simulink model "ss2tf_model"  (R2018b)
settings: Solver=VariableStepAuto  StartTime=0.0  StopTime=600  RelTol=1e-3
undefined symbols (not defined in the file or in its folder): filteredInvTF, heave, seaWave, SS_full, surge
settings Model: Creator=user  LastModifiedBy=user

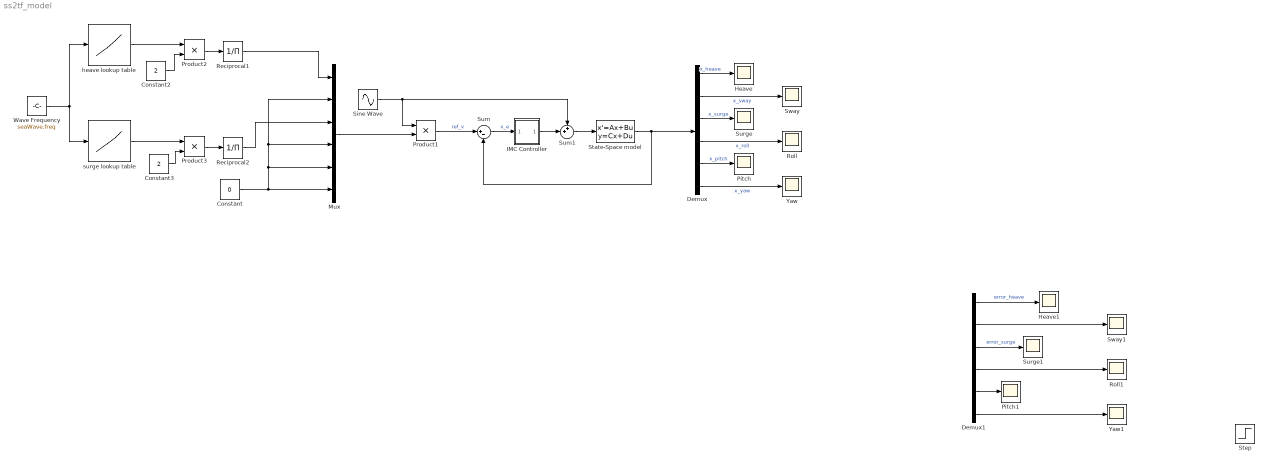
== system ss2tf_model ==
  Constant : Constant  Value=0
  Constant2 : Constant  Value=2
  Constant3 : Constant  Value=2
  Demux : Demux  Outputs=6
  Demux1 : Demux  Outputs=6
  Heave : Scope
  Heave1 : Scope
  IMC Controller : Subsystem
      mask Display: fprintf("K")
  Mux : Mux  Inputs=6
  Pitch : Scope
  Pitch1 : Scope
  Product1 : Product
  Product2 : Product
  Product3 : Product
  Reciprocal1 : Product  Inputs=/
  Reciprocal2 : Product  Inputs=/
  Roll : Scope
  Roll1 : Scope
  Sine Wave : Sin  Amplitude=seaWave.amp  Frequency=seaWave.freq  SampleTime=0
  State-Space model : StateSpace  A=SS_full.A  B=SS_full.B  C=SS_full.C  D=SS_full.D  InitialCondition=0
  Step : Step  Time=20  SampleTime=0
  Sum : Sum  Inputs=|+-
  Sum1 : Sum  Inputs=++|
  Surge : Scope
  Surge1 : Scope
  Sway : Scope
  Sway1 : Scope
  Wave Frequency : Constant  Value=seaWave.freq
  Yaw : Scope
  Yaw1 : Scope
  heave lookup table : Lookup_n-D  NumberOfTableDimensions=1  BreakpointsForDimension1=heave.freq  Table=heave.amp  InternalRulePriority=Speed  RndMeth=Simplest  InputSameDT=on
  surge lookup table : Lookup_n-D  NumberOfTableDimensions=1  BreakpointsForDimension1=surge.freq  Table=surge.amp  InternalRulePriority=Speed  RndMeth=Simplest  InputSameDT=on
  wires:
  Wave Frequency/1 -> heave lookup table/1, surge lookup table/1
  Constant/1 -> Mux/2, Mux/4, Mux/5, Mux/6
  Mux/1 -> Product1/2
  Product1/1 -> Sum/1  "ref_v"
  Sine Wave/1 -> Sum1/1, Product1/1
  Demux/1 -> Heave/1  "x_heave"
  Demux/3 -> Surge/1  "x_surge"
  Demux/5 -> Pitch/1  "x_pitch"
  Sum1/1 -> State-Space model/1
  Sum/1 -> IMC Controller/1(x_e)  "x_e"
  IMC Controller/1(control signal) -> Sum1/2
  Demux/2 -> Sway/1  "x_sway"
  Demux/4 -> Roll/1  "x_roll"
  Demux/6 -> Yaw/1  "x_yaw"
  heave lookup table/1 -> Product2/1
  Constant2/1 -> Product2/2
  Product2/1 -> Reciprocal1/1
  Reciprocal1/1 -> Mux/1
  surge lookup table/1 -> Product3/1
  Constant3/1 -> Product3/2
  Product3/1 -> Reciprocal2/1
  Reciprocal2/1 -> Mux/3
  Demux1/6 -> Yaw1/1
  Demux1/5 -> Pitch1/1
  Demux1/2 -> Sway1/1
  Demux1/4 -> Roll1/1
  Demux1/3 -> Surge1/1  "error_surge"
  Demux1/1 -> Heave1/1  "error_heave"
  State-Space model/1 -> Demux/1, Sum/2

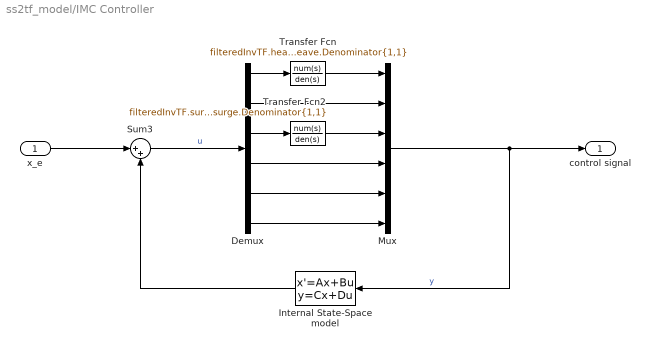
== system ss2tf_model/IMC Controller ==
  x_e : Inport
  Demux : Demux  Outputs=6
  Internal State-Space model : StateSpace  A=SS_full.A  B=SS_full.B  C=SS_full.C  D=SS_full.D  InitialCondition=0
  Mux : Mux  Inputs=6
  Sum3 : Sum  Inputs=|++
  Transfer Fcn : TransferFcn  Numerator=filteredInvTF.heave.Numerator{1,1}  Denominator=filteredInvTF.heave.Denominator{1,1}
  Transfer Fcn2 : TransferFcn  Numerator=filteredInvTF.surge.Numerator{1,1}  Denominator=filteredInvTF.surge.Denominator{1,1}
  control signal : Outport
  wires:
  Sum3/1 -> Demux/1  "u"
  Demux/1 -> Transfer Fcn/1
  Internal State-Space model/1 -> Sum3/2
  Demux/3 -> Transfer Fcn2/1
  Transfer Fcn/1 -> Mux/1
  Mux/1 -> Internal State-Space model/1, control signal/1  "y"
  Transfer Fcn2/1 -> Mux/3
  Demux/2 -> Mux/2
  Demux/4 -> Mux/4
  Demux/5 -> Mux/5
  Demux/6 -> Mux/6
  x_e/1 -> Sum3/1
